simulink model "Modelo8_Harness2"  (R2020b)
settings: Solver=FixedStepAuto  StartTime=0.0  StopTime=inf  FixedStep=1e-2  MaxStep=1e-4  RelTol=1e-3
settings Model: Creator=GoniR  LastModifiedBy=GoniR
settings SolverCC: ConcurrentTasks=on  ZeroCrossAlgorithm=Adaptive  AutoInsertRateTranBlk=on
settings DebuggingCC: MaskedZcDiagnostic=none  IgnoredZcDiagnostic=none
settings HardwareCC: ProdHWDeviceType=AMD->x86-64 (Windows64)
settings SFSimCC: SimTargetLang=C++
settings ConfigComp: PLC_TargetIDE=codesys23

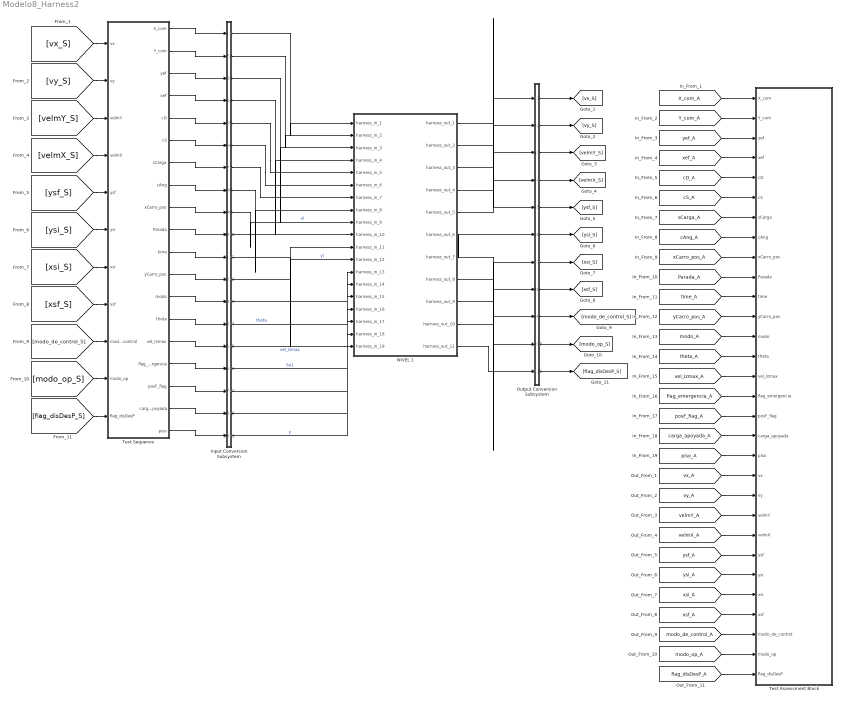
== system Modelo8_Harness2 ==
  Input Conversion Subsystem : Subsystem  Tag=__SLT_ICS__  Description=|
      | Signal spec.
      | and routing
      settings: AttributesFormatString=%<Description>
  NIVEL 1 : Subsystem  Tag=__SL_testing_harness_stub_
  Output Conversion Subsystem : Subsystem  Tag=__SLT_OCS__  Description=|
      | Signal spec.
      | and routing
      settings: AttributesFormatString=%<Description>
  Test Assessment Block : Test Sequence  Tag=__SLT_ASMT__  TreatAsAtomicUnit=on
  Test Sequence : Test Sequence  TreatAsAtomicUnit=on
  wires:
  [X_com_A] -> Test Assessment Block/1(X_com)
  [Y_com_A] -> Test Assessment Block/2(Y_com)
  [yef_A] -> Test Assessment Block/3(yef)
  [xef_A] -> Test Assessment Block/4(xef)
  [cD_A] -> Test Assessment Block/5(cD)
  [cS_A] -> Test Assessment Block/6(cS)
  [sCarga_A] -> Test Assessment Block/7(sCarga)
  [cAng_A] -> Test Assessment Block/8(cAng)
  [xCarro_pos_A] -> Test Assessment Block/9(xCarro_pos)
  [Parada_A] -> Test Assessment Block/10(Parada)
  [time_A] -> Test Assessment Block/11(time)
  [yCarro_pos_A] -> Test Assessment Block/12(yCarro_pos)
  [modo_A] -> Test Assessment Block/13(modo)
  [theta_A] -> Test Assessment Block/14(theta)
  [vel_Izmax_A] -> Test Assessment Block/15(vel_Izmax)
  [flag_emergencia_A] -> Test Assessment Block/16(flag_emergencia)
  [posF_flag_A] -> Test Assessment Block/17(posF_flag)
  [carga_apoyada_A] -> Test Assessment Block/18(carga_apoyada)
  [piso_A] -> Test Assessment Block/19(piso)
  [vx_A] -> Test Assessment Block/20(vx)
  [vy_A] -> Test Assessment Block/21(vy)
  [velmY_A] -> Test Assessment Block/22(velmY)
  [velmX_A] -> Test Assessment Block/23(velmX)
  [ysf_A] -> Test Assessment Block/24(ysf)
  [ysi_A] -> Test Assessment Block/25(ysi)
  [xsi_A] -> Test Assessment Block/26(xsi)
  [xsf_A] -> Test Assessment Block/27(xsf)
  [modo_de_control_A] -> Test Assessment Block/28(modo_de_control)
  [modo_op_A] -> Test Assessment Block/29(modo_op)
  [flag_disDesP_A] -> Test Assessment Block/30(flag_disDesP)
  Test Sequence/1(X_com) -> Input Conversion Subsystem/1(Inport_1)
  Test Sequence/2(Y_com) -> Input Conversion Subsystem/2(Inport_2)
  Test Sequence/3(yef) -> Input Conversion Subsystem/3(Inport_3)
  Test Sequence/4(xef) -> Input Conversion Subsystem/4(Inport_4)
  Test Sequence/5(cD) -> Input Conversion Subsystem/5(Inport_5)
  Test Sequence/6(cS) -> Input Conversion Subsystem/6(Inport_6)
  Test Sequence/7(sCarga) -> Input Conversion Subsystem/7(Inport_7)
  Test Sequence/8(cAng) -> Input Conversion Subsystem/8(Inport_8)
  Test Sequence/9(xCarro_pos) -> Input Conversion Subsystem/9(Inport_9)
  Test Sequence/10(Parada) -> Input Conversion Subsystem/10(Inport_10)
  Test Sequence/11(time) -> Input Conversion Subsystem/11(Inport_11)
  Test Sequence/12(yCarro_pos) -> Input Conversion Subsystem/12(Inport_12)
  Test Sequence/13(modo) -> Input Conversion Subsystem/13(Inport_13)
  Test Sequence/14(theta) -> Input Conversion Subsystem/14(Inport_14)
  Test Sequence/15(vel_Izmax) -> Input Conversion Subsystem/15(Inport_15)
  Test Sequence/16(flag_emergencia) -> Input Conversion Subsystem/16(Inport_16)
  Test Sequence/17(posF_flag) -> Input Conversion Subsystem/17(Inport_17)
  Test Sequence/18(carga_apoyada) -> Input Conversion Subsystem/18(Inport_18)
  Test Sequence/19(piso) -> Input Conversion Subsystem/19(Inport_19)
  [vx_S] -> Test Sequence/1(vx)
  [vy_S] -> Test Sequence/2(vy)
  [velmY_S] -> Test Sequence/3(velmY)
  [velmX_S] -> Test Sequence/4(velmX)
  [ysf_S] -> Test Sequence/5(ysf)
  [ysi_S] -> Test Sequence/6(ysi)
  [xsi_S] -> Test Sequence/7(xsi)
  [xsf_S] -> Test Sequence/8(xsf)
  [modo_de_control_S] -> Test Sequence/9(modo_de_control)
  [modo_op_S] -> Test Sequence/10(modo_op)
  [flag_disDesP_S] -> Test Sequence/11(flag_disDesP)
  Output Conversion Subsystem/1(Outport_1) -> [vx_S]
  Output Conversion Subsystem/2(Outport_2) -> [vy_S]
  Output Conversion Subsystem/3(Outport_3) -> [velmY_S]
  Output Conversion Subsystem/4(Outport_4) -> [velmX_S]
  Output Conversion Subsystem/5(Outport_5) -> [ysf_S]
  Output Conversion Subsystem/6(Outport_6) -> [ysi_S]
  Output Conversion Subsystem/7(Outport_7) -> [xsi_S]
  Output Conversion Subsystem/8(Outport_8) -> [xsf_S]
  Output Conversion Subsystem/9(Outport_9) -> [modo_de_control_S]
  Output Conversion Subsystem/10(Outport_10) -> [modo_op_S]
  Output Conversion Subsystem/11(Outport_11) -> [flag_disDesP_S]
  Input Conversion Subsystem/1(Outport_1) -> NIVEL 1/1(harness_in_1)
  Input Conversion Subsystem/2(Outport_2) -> NIVEL 1/2(harness_in_2)
  Input Conversion Subsystem/3(Outport_3) -> NIVEL 1/3(harness_in_3)
  Input Conversion Subsystem/4(Outport_4) -> NIVEL 1/4(harness_in_4)
  Input Conversion Subsystem/5(Outport_5) -> NIVEL 1/5(harness_in_5)
  Input Conversion Subsystem/6(Outport_6) -> NIVEL 1/6(harness_in_6)
  Input Conversion Subsystem/7(Outport_7) -> NIVEL 1/7(harness_in_7)
  Input Conversion Subsystem/8(Outport_8) -> NIVEL 1/8(harness_in_8)
  Input Conversion Subsystem/9(Outport_9) -> NIVEL 1/9(harness_in_9)  "xl"
  Input Conversion Subsystem/10(Outport_10) -> NIVEL 1/10(harness_in_10)
  Input Conversion Subsystem/11(Outport_11) -> NIVEL 1/11(harness_in_11)
  Input Conversion Subsystem/12(Outport_12) -> NIVEL 1/12(harness_in_12)  "yl"
  Input Conversion Subsystem/13(Outport_13) -> NIVEL 1/13(harness_in_13)
  Input Conversion Subsystem/14(Outport_14) -> NIVEL 1/14(harness_in_14)  "theta"
  Input Conversion Subsystem/15(Outport_15) -> NIVEL 1/15(harness_in_15)  "vel_Izmax"
  Input Conversion Subsystem/16(Outport_16) -> NIVEL 1/16(harness_in_16)  "Se1"
  Input Conversion Subsystem/17(Outport_17) -> NIVEL 1/17(harness_in_17)
  Input Conversion Subsystem/18(Outport_18) -> NIVEL 1/18(harness_in_18)
  Input Conversion Subsystem/19(Outport_19) -> NIVEL 1/19(harness_in_19)  "y"
  NIVEL 1/1(harness_out_1) -> Output Conversion Subsystem/1(Inport_1)
  NIVEL 1/2(harness_out_2) -> Output Conversion Subsystem/2(Inport_2)
  NIVEL 1/3(harness_out_3) -> Output Conversion Subsystem/3(Inport_3)
  NIVEL 1/4(harness_out_4) -> Output Conversion Subsystem/4(Inport_4)
  NIVEL 1/5(harness_out_5) -> Output Conversion Subsystem/5(Inport_5)
  NIVEL 1/6(harness_out_6) -> Output Conversion Subsystem/6(Inport_6)
  NIVEL 1/7(harness_out_7) -> Output Conversion Subsystem/7(Inport_7)
  NIVEL 1/8(harness_out_8) -> Output Conversion Subsystem/8(Inport_8)
  NIVEL 1/9(harness_out_9) -> Output Conversion Subsystem/9(Inport_9)
  NIVEL 1/10(harness_out_10) -> Output Conversion Subsystem/10(Inport_10)
  NIVEL 1/11(harness_out_11) -> Output Conversion Subsystem/11(Inport_11)

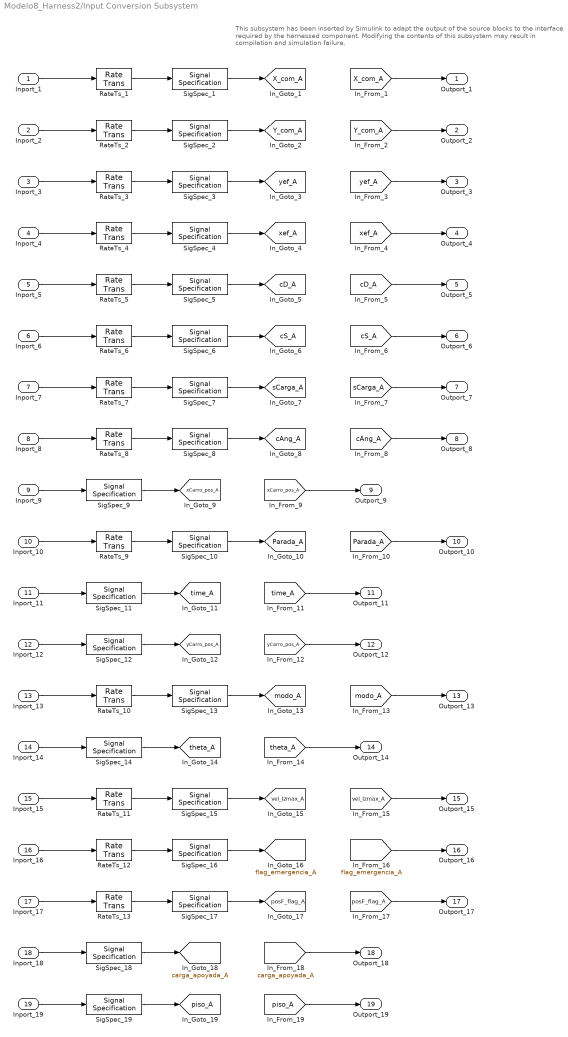
== system Modelo8_Harness2/Input Conversion Subsystem ==
  note: This subsystem has been inserted by Simulink to adapt the output of the source blocks to the interface required by the harnessed component.
      |  Modifying the contents of this subsystem may result in compilation and simulation failure.
  Inport_1 : Inport
  Inport_2 : Inport  Port=2
  Inport_3 : Inport  Port=3
  Inport_4 : Inport  Port=4
  Inport_5 : Inport  Port=5
  Inport_6 : Inport  Port=6
  Inport_7 : Inport  Port=7
  Inport_8 : Inport  Port=8
  Inport_9 : Inport  Port=9
  Inport_10 : Inport  Port=10
  Inport_11 : Inport  Port=11
  Inport_12 : Inport  Port=12
  Inport_13 : Inport  Port=13
  Inport_14 : Inport  Port=14
  Inport_15 : Inport  Port=15
  Inport_16 : Inport  Port=16
  Inport_17 : Inport  Port=17
  Inport_18 : Inport  Port=18
  Inport_19 : Inport  Port=19
  RateTs_{1..2,5..6,9..12} (8 alike) : RateTransition  OutPortSampleTime=0.01
  RateTs_{3..4,7..8,13} (5 alike) : RateTransition  OutPortSampleTime=[-1, 0]
  SigSpec_{1..2,5..6,10,13,15..16} (8 alike) : SignalSpecification  OutDataTypeStr=double  Dimensions=[1]  SampleTime=0.01
  SigSpec_{3..4,7..9,11..12,14,17..19} (11 alike) : SignalSpecification  OutDataTypeStr=double  Dimensions=[1]  SampleTime=[-1, 0]
  Outport_1 : Outport
  Outport_2 : Outport  Port=2
  Outport_3 : Outport  Port=3
  Outport_4 : Outport  Port=4
  Outport_5 : Outport  Port=5
  Outport_6 : Outport  Port=6
  Outport_7 : Outport  Port=7
  Outport_8 : Outport  Port=8
  Outport_9 : Outport  Port=9
  Outport_10 : Outport  Port=10
  Outport_11 : Outport  Port=11
  Outport_12 : Outport  Port=12
  Outport_13 : Outport  Port=13
  Outport_14 : Outport  Port=14
  Outport_15 : Outport  Port=15
  Outport_16 : Outport  Port=16
  Outport_17 : Outport  Port=17
  Outport_18 : Outport  Port=18
  Outport_19 : Outport  Port=19
  tag scope: Parada_A=global, X_com_A=global, Y_com_A=global, cAng_A=global, cD_A=global, cS_A=global, carga_apoyada_A=global, flag_emergencia_A=global, modo_A=global, piso_A=global, posF_flag_A=global, sCarga_A=global, theta_A=global, time_A=global, vel_Izmax_A=global, xCarro_pos_A=global, xef_A=global, yCarro_pos_A=global, yef_A=global
  wires:
  [X_com_A] -> Outport_1/1
  SigSpec_1/1 -> [X_com_A]
  RateTs_1/1 -> SigSpec_1/1
  Inport_1/1 -> RateTs_1/1
  [Y_com_A] -> Outport_2/1
  SigSpec_2/1 -> [Y_com_A]
  RateTs_2/1 -> SigSpec_2/1
  Inport_2/1 -> RateTs_2/1
  [yef_A] -> Outport_3/1
  SigSpec_3/1 -> [yef_A]
  RateTs_3/1 -> SigSpec_3/1
  Inport_3/1 -> RateTs_3/1
  [xef_A] -> Outport_4/1
  SigSpec_4/1 -> [xef_A]
  RateTs_4/1 -> SigSpec_4/1
  Inport_4/1 -> RateTs_4/1
  [cD_A] -> Outport_5/1
  SigSpec_5/1 -> [cD_A]
  RateTs_5/1 -> SigSpec_5/1
  Inport_5/1 -> RateTs_5/1
  [cS_A] -> Outport_6/1
  SigSpec_6/1 -> [cS_A]
  RateTs_6/1 -> SigSpec_6/1
  Inport_6/1 -> RateTs_6/1
  [sCarga_A] -> Outport_7/1
  SigSpec_7/1 -> [sCarga_A]
  RateTs_7/1 -> SigSpec_7/1
  Inport_7/1 -> RateTs_7/1
  [cAng_A] -> Outport_8/1
  SigSpec_8/1 -> [cAng_A]
  RateTs_8/1 -> SigSpec_8/1
  Inport_8/1 -> RateTs_8/1
  [xCarro_pos_A] -> Outport_9/1
  SigSpec_9/1 -> [xCarro_pos_A]
  Inport_9/1 -> SigSpec_9/1
  [Parada_A] -> Outport_10/1
  SigSpec_10/1 -> [Parada_A]
  RateTs_9/1 -> SigSpec_10/1
  Inport_10/1 -> RateTs_9/1
  [time_A] -> Outport_11/1
  SigSpec_11/1 -> [time_A]
  Inport_11/1 -> SigSpec_11/1
  [yCarro_pos_A] -> Outport_12/1
  SigSpec_12/1 -> [yCarro_pos_A]
  Inport_12/1 -> SigSpec_12/1
  [modo_A] -> Outport_13/1
  SigSpec_13/1 -> [modo_A]
  RateTs_10/1 -> SigSpec_13/1
  Inport_13/1 -> RateTs_10/1
  [theta_A] -> Outport_14/1
  SigSpec_14/1 -> [theta_A]
  Inport_14/1 -> SigSpec_14/1
  [vel_Izmax_A] -> Outport_15/1
  SigSpec_15/1 -> [vel_Izmax_A]
  RateTs_11/1 -> SigSpec_15/1
  Inport_15/1 -> RateTs_11/1
  [flag_emergencia_A] -> Outport_16/1
  SigSpec_16/1 -> [flag_emergencia_A]
  RateTs_12/1 -> SigSpec_16/1
  Inport_16/1 -> RateTs_12/1
  [posF_flag_A] -> Outport_17/1
  SigSpec_17/1 -> [posF_flag_A]
  RateTs_13/1 -> SigSpec_17/1
  Inport_17/1 -> RateTs_13/1
  [carga_apoyada_A] -> Outport_18/1
  SigSpec_18/1 -> [carga_apoyada_A]
  Inport_18/1 -> SigSpec_18/1
  [piso_A] -> Outport_19/1
  SigSpec_19/1 -> [piso_A]
  Inport_19/1 -> SigSpec_19/1

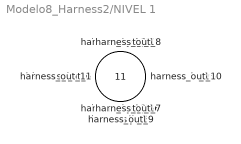
== system Modelo8_Harness2/NIVEL 1 ==
  harness_in_1 : Inport
  harness_in_2 : Inport  Port=2
  harness_in_3 : Inport  Port=3
  harness_in_4 : Inport  Port=4
  harness_in_5 : Inport  Port=5
  harness_in_6 : Inport  Port=6
  harness_in_7 : Inport  Port=7
  harness_in_8 : Inport  Port=8
  harness_in_9 : Inport  Port=9
  harness_in_10 : Inport  Port=10
  harness_in_11 : Inport  Port=11
  harness_in_12 : Inport  Port=12
  harness_in_13 : Inport  Port=13
  harness_in_14 : Inport  Port=14
  harness_in_15 : Inport  Port=15
  harness_in_16 : Inport  Port=16
  harness_in_17 : Inport  Port=17
  harness_in_18 : Inport  Port=18
  harness_in_19 : Inport  Port=19
  harness_out_1 : Outport
  harness_out_2 : Outport  Port=2
  harness_out_3 : Outport  Port=3
  harness_out_4 : Outport  Port=4
  harness_out_5 : Outport  Port=5
  harness_out_6 : Outport  Port=6
  harness_out_7 : Outport  Port=7
  harness_out_8 : Outport  Port=8
  harness_out_9 : Outport  Port=9
  harness_out_10 : Outport  Port=10
  harness_out_11 : Outport  Port=11

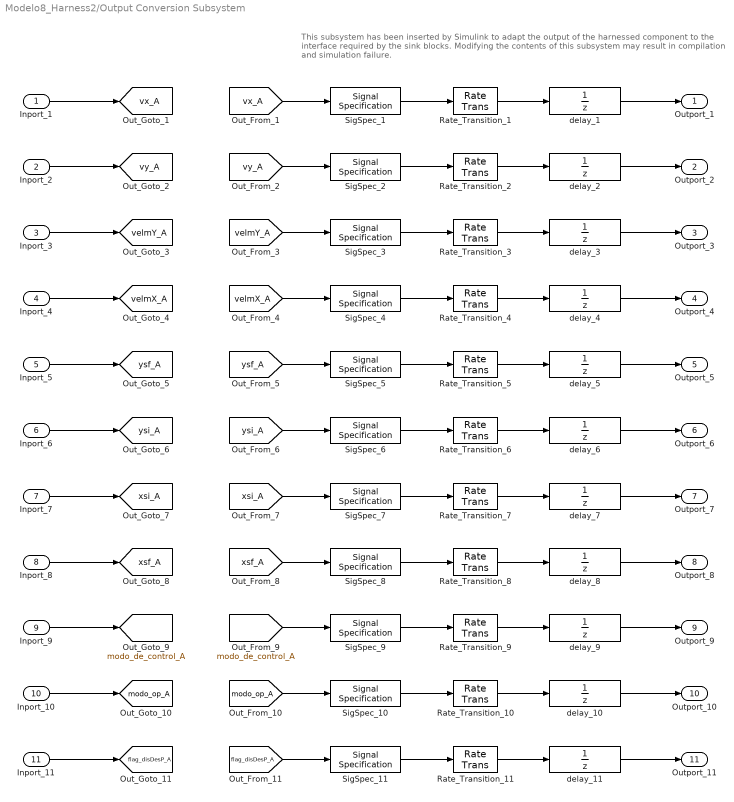
== system Modelo8_Harness2/Output Conversion Subsystem ==
  note: This subsystem has been inserted by Simulink to adapt the output of the harnessed component to the interface required by the sink blocks.
      |  Modifying the contents of this subsystem may result in compilation and simulation failure.
  Inport_1 : Inport
  Inport_2 : Inport  Port=2
  Inport_3 : Inport  Port=3
  Inport_4 : Inport  Port=4
  Inport_5 : Inport  Port=5
  Inport_6 : Inport  Port=6
  Inport_7 : Inport  Port=7
  Inport_8 : Inport  Port=8
  Inport_9 : Inport  Port=9
  Inport_10 : Inport  Port=10
  Inport_11 : Inport  Port=11
  Rate_Transition_{1..11} (11 alike) : RateTransition  OutPortSampleTimeOpt=Inherit
  SigSpec_{1..8,10..11} (10 alike) : SignalSpecification  OutDataTypeStr=double  Dimensions=[1]  SampleTime=0.01
  SigSpec_9 : SignalSpecification  OutDataTypeStr=double  Dimensions=[1, 1]  SampleTime=0.01
  delay_{1..11} (11 alike) : UnitDelay  SampleTime=-1
  Outport_1 : Outport
  Outport_2 : Outport  Port=2
  Outport_3 : Outport  Port=3
  Outport_4 : Outport  Port=4
  Outport_5 : Outport  Port=5
  Outport_6 : Outport  Port=6
  Outport_7 : Outport  Port=7
  Outport_8 : Outport  Port=8
  Outport_9 : Outport  Port=9
  Outport_10 : Outport  Port=10
  Outport_11 : Outport  Port=11
  tag scope: flag_disDesP_A=global, modo_de_control_A=global, modo_op_A=global, velmX_A=global, velmY_A=global, vx_A=global, vy_A=global, xsf_A=global, xsi_A=global, ysf_A=global, ysi_A=global
  wires:
  Inport_1/1 -> [vx_A]
  [vx_A] -> SigSpec_1/1
  SigSpec_1/1 -> Rate_Transition_1/1
  Rate_Transition_1/1 -> delay_1/1
  delay_1/1 -> Outport_1/1
  Inport_2/1 -> [vy_A]
  [vy_A] -> SigSpec_2/1
  SigSpec_2/1 -> Rate_Transition_2/1
  Rate_Transition_2/1 -> delay_2/1
  delay_2/1 -> Outport_2/1
  Inport_3/1 -> [velmY_A]
  [velmY_A] -> SigSpec_3/1
  SigSpec_3/1 -> Rate_Transition_3/1
  Rate_Transition_3/1 -> delay_3/1
  delay_3/1 -> Outport_3/1
  Inport_4/1 -> [velmX_A]
  [velmX_A] -> SigSpec_4/1
  SigSpec_4/1 -> Rate_Transition_4/1
  Rate_Transition_4/1 -> delay_4/1
  delay_4/1 -> Outport_4/1
  Inport_5/1 -> [ysf_A]
  [ysf_A] -> SigSpec_5/1
  SigSpec_5/1 -> Rate_Transition_5/1
  Rate_Transition_5/1 -> delay_5/1
  delay_5/1 -> Outport_5/1
  Inport_6/1 -> [ysi_A]
  [ysi_A] -> SigSpec_6/1
  SigSpec_6/1 -> Rate_Transition_6/1
  Rate_Transition_6/1 -> delay_6/1
  delay_6/1 -> Outport_6/1
  Inport_7/1 -> [xsi_A]
  [xsi_A] -> SigSpec_7/1
  SigSpec_7/1 -> Rate_Transition_7/1
  Rate_Transition_7/1 -> delay_7/1
  delay_7/1 -> Outport_7/1
  Inport_8/1 -> [xsf_A]
  [xsf_A] -> SigSpec_8/1
  SigSpec_8/1 -> Rate_Transition_8/1
  Rate_Transition_8/1 -> delay_8/1
  delay_8/1 -> Outport_8/1
  Inport_9/1 -> [modo_de_control_A]
  [modo_de_control_A] -> SigSpec_9/1
  SigSpec_9/1 -> Rate_Transition_9/1
  Rate_Transition_9/1 -> delay_9/1
  delay_9/1 -> Outport_9/1
  Inport_10/1 -> [modo_op_A]
  [modo_op_A] -> SigSpec_10/1
  SigSpec_10/1 -> Rate_Transition_10/1
  Rate_Transition_10/1 -> delay_10/1
  delay_10/1 -> Outport_10/1
  Inport_11/1 -> [flag_disDesP_A]
  [flag_disDesP_A] -> SigSpec_11/1
  SigSpec_11/1 -> Rate_Transition_11/1
  Rate_Transition_11/1 -> delay_11/1
  delay_11/1 -> Outport_11/1

== stateflow chart Modelo8_Harness2/Test Assessment Block ==
  settings: stateMachineType=SIMPLIFIED_MACHINE
  state Run
    state step_1_1
    state step_1_2
    (default) -> (junction 22)
    Run -> (junction 22)
    (junction 22) -> (junction 23) [order 1] : [t < 5]
    (junction 23) -> step_1_1 [order 1] : [~in(step_1_1)]
    (junction 23) -> (junction 26) [order 2]
    (junction 31) -> (junction 32)
    (junction 32) -> step_1_2 [order 1] : [~in(step_1_2)]
    (junction 32) -> (junction 35) [order 2]
    (junction 22) -> (junction 31) [order 2]
  (default) -> Run
  data: X_com input double size=[1]; Y_com input double size=[1]; yef input double size=[1]; xef input double size=[1]; cD input double size=[1]; cS input double size=[1]; sCarga input double size=[1]; cAng input double size=[1]; xCarro_pos input double size=[1]; Parada input double size=[1]; time input double size=[1]; yCarro_pos input double size=[1]; modo input double size=[1]; theta input double size=[1]; vel_Izmax input double size=[1]; flag_emergencia input double size=[1]; posF_flag input double size=[1]; carga_apoyada input double size=[1]; piso input double size=[1]; vx input double size=[1]; vy input double size=[1]; velmY input double size=[1]; velmX input double size=[1]; ysf input double size=[1]; ysi input double size=[1]; xsi input double size=[1]; xsf input double size=[1]; modo_de_control input double size=[1, 1]; modo_op input double size=[1]; flag_disDesP input double size=[1]

== stateflow chart Modelo8_Harness2/Test Sequence ==
  settings: updateMethod=DISCRETE  sampleTime=0.01  stateMachineType=SIMPLIFIED_MACHINE
  state Run
    %% Initialize data outputs.
    X_com = 0;
    Y_com = 0;
    yef = 0;
    xef = 0;
    cD = 0;
    cS = 0;
    sCarga = 0;
    cAng = 0;
    xCarro_pos = 0;
    Parada = 0;
    time = 0;
    yCarro_pos = 0;
    modo = 0;
    theta = 0;
    vel_Izmax = 0;
    flag_emergencia = 0;
    posF_flag = 0;
    carga_apoyada = 0;
    piso = 0;
  (default) -> Run
  data: vx input double size=[1]; vy input double size=[1]; velmY input double size=[1]; velmX input double size=[1]; ysf input double size=[1]; ysi input double size=[1]; xsi input double size=[1]; xsf input double size=[1]; modo_de_control input double size=[1, 1]; modo_op input double size=[1]; flag_disDesP input double size=[1]; X_com output double size=[1]; Y_com output double size=[1]; yef output double size=[1]; xef output double size=[1]; cD output double size=[1]; cS output double size=[1]; sCarga output double size=[1]; cAng output double size=[1]; xCarro_pos output double size=[1]; Parada output double size=[1]; time output double size=[1]; yCarro_pos output double size=[1]; modo output double size=[1]; theta output double size=[1]; vel_Izmax output double size=[1]; flag_emergencia output double size=[1]; posF_flag output double size=[1]; carga_apoyada output double size=[1]; piso output double size=[1]
